simulink model "DrivetrainEv"  (R2020a)
settings: Solver=VariableStepAuto  StartTime=0.0  StopTime=2474  RelTol=1e-3  EnableMultiTasking=on
model workspace (MAT data in the model file):
  Af = 2.27
  Bx = 10
  Cd = 0.28
  Cl = 0.1
  Cpm = 0.1
  Cx = 1.65
  Dx = 1
  Ex = 0.01
  FZMAX = 6570
  FZMIN = 0
  Fc = 500
  FsbF = [-700000 -7000 -700 0 700 7000 700000]
  FsbR = [-700000 -7000 -700 0 700 7000 700000]
  FskF = [-8928.57142857 -178.571428571 0 357.142857143 535.714285714 9285.71428571]
  FskR = [-5357.14285714 -107.142857143 0 214.285714286 321.428571429 5571.42857143]
  Iyy = 3000
  Iyy_Whl = 0.8
  J = 0.01
  Jd = 0.025
  Jmotor = 0.023
  Jw1 = 0.01
  Jw2 = 0.01
  Lrel = 0.15
  Mass = 235.45
  NF = 2
  NR = 2
  Ndiff = 7.94
  Ndisks = 4
  Pabs = 101325
  Re = 0.203
  Reff_LSD = 0.2
  Rm = 0.15
  T = 273
  UNLOADED_RADIUS = 0.206
  VXLOW = 2
  aMy = 0.01
  a_CG = 1.188
  alphaMy = 0
  b = Simulink.Parameter
  b.Value = 400
  b.DataType = 'auto'
  b.Dimensions = [1 1]
  b1 = 100
  bMy = 0
  b_CG = 1.512
  b_J = 0.001
  bd = 0.001
  betaMy = 1
  br = 0.001
  bw1 = 0.001
  bw2 = 0.001
  cMy = 0
  disk_abore = 0.05
  domega_o = 0
  dw = [0 10 20 40 60 80 100]
  dzdotsF = [-10 -1 -0.1 0 0.1 1 10]
  dzdotsR = [-10 -1 -0.1 0 0.1 1 10]
  dzsF = [-0.005 -0.0001 0 0.2 0.2001 0.2051]
  dzsR = [-0.005 -0.0001 0 0.2 0.2001 0.2051]
  g = 9.81
  h = 0.5
  k = Simulink.Parameter
  k.Value = 10000
  k.DataType = 'auto'
  k.Dimensions = [1 1]
  k1 = 50000
  kappamax = 1.5
  lam_x = 1
  mu_kinetic = 0.35
  mu_static = 0.45
  muc = [0.16 0.13 0.115 0.11 0.105 0.1025 0.10125]
  num_pads = 2
  omega1_c = 3000
  omega_c = Simulink.Parameter
  omega_c.Value = 100
  omega_c.DataType = 'auto'
  omega_c.Dimensions = [1 1]
  omega_o = 0
  omega_o_J = 0
  omegao = 0
  omegaw1o = 0
  omegaw2o = 0
  press = 234400
  q_o = 0
  tauC_LSD = 0.01
  theta_o = 0
  theta_o_Veh = 0
  wc_shaft = Simulink.Parameter
  wc_shaft.Value = 0.1
  wc_shaft.DataType = 'auto'
  wc_shaft.Dimensions = [1 1]
  x_o = 0
  xdot_o = 0
  z_o = -0.35
  zdot_o = 0
libraries: autolibsharedcoupling x7, autolibpowerinfoutils x6, autolibshareddiff x4, autolibshared x3, autolibcoupling x1
(part 1 of 3)
settings Model: ModifiedByFormat=The MathWorks, Inc.  SimulationMode=rapid-accelerator  PauseTimes=10  Creator=The MathWorks, Inc.  LastModifiedBy=The MathWorks, Inc.
settings SolverCC: DecoupledContinuousIntegration=on  MinimalZcImpactIntegration=on
settings DataIOCC: DSMLogging=off  ReturnWorkspaceOutputs=off
settings DebuggingCC: MergeDetectMultiDrivingBlocksExec=none  PregeneratedLibrarySubsystemCodeDiagnostic=none  ArithmeticOperatorsInVariantConditions=warning
settings ModelReferenceCC: PropagateSignalLabelsOutOfModel=off
settings SFSimCC: SimUseLocalCustomCode=off
settings RTWCC: RTWUseLocalCustomCode=off
settings CodeAppCC: StateflowObjectComments=on
settings GRTTargetCC: TargetLangStandard=C89/C90 (ANSI)
settings ConfigComp: CovMetricSettings=dsw  CovHtmlReporting=on  CovSaveCumulativeToWorkspaceVar=on  CovSaveSingleToWorkspaceVar=on  CovShowResultsExplorer=off  CovExternalEMLEnable=off
settings SimscapeCC: SimscapeNormalizeSystem=off

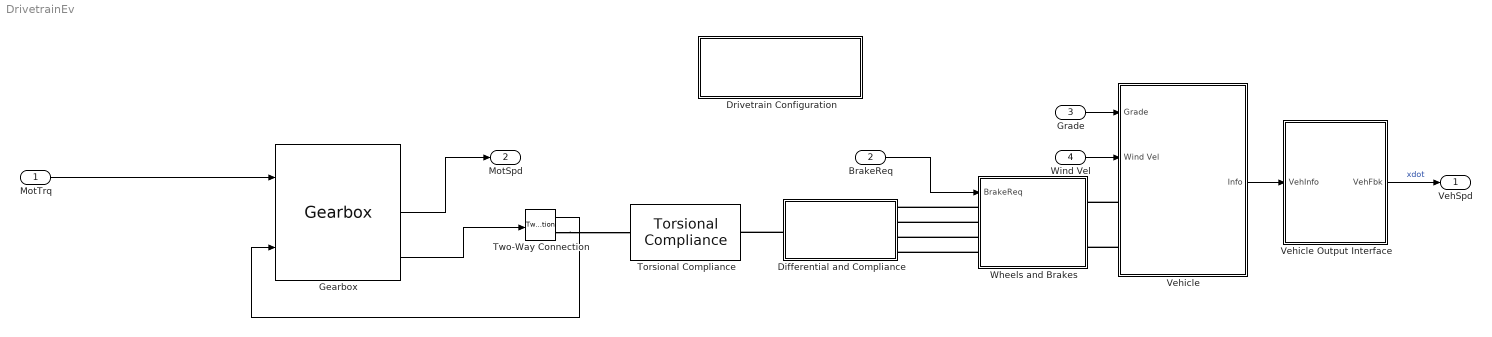
== system DrivetrainEv ==
  MotTrq : Inport
  BrakeReq : Inport  Port=2
  Grade : Inport  Port=3
  Wind Vel : Inport  Port=4
  Differential and Compliance : Subsystem  Variant=on  VariantControlMode=Label  LabelModeActiveChoice=1
  Drivetrain Configuration : Subsystem  mask(Drivetrain Configuration){drivetrainMode=Rear Wheel Drive}
      mask prompts: drivetrainMode "Drivetrain Mode"
      mask help: Use this block to configure the dirvetrain mode.
      settings: AttributesFormatString=Active Mode: %<drivetrainMode>
      mask TypeOptions drivetrainMode: Front Wheel Drive | Rear Wheel Drive | All Wheel Drive
      mask Callback drivetrainMode:
      | switch get_param(gcb,'drivetrainMode')
      |     case 'Front Wheel Drive'
      |         set_param([bdroot '/Differential and Compliance'],'OverrideUsingVariant','0')
      |     case 'Rear Wheel Drive'
      |         set_param([bdroot '/Differential and Compliance'],'OverrideUsingVariant','1')
      |     case 'All Wheel Drive'
      |         set_param([bdroot '/Differential and Compliance'],'OverrideUsingVariant','2')
      |     otherwise
      |         set_param([bdroot '/Differential and Compliance'],'OverrideUsingVariant','0')
      | end
      mask Display: disp('Double click to configure drivetrain')
  Gearbox : autolibcoupling/Gearbox  port_config=Simulink  input_config=Torque input - velocity output  DiffEffModelPopup=Constant  InterpMethod=Flat  dirSwitch=on  extTamb=off  N=9/40  J1=.023  J2=.023  b1=0  b2=0  theta1_o=0  w1_o=0  eta=1  eta_tbl=reshape([0.64 0.76 0.8 0.81 0.83 0.84 0.84 0.56 0.73 0.78 0.8 0.83 0.84 0.84 0.54 0.71 0.77 0.8 0.82 0.84 0.84 0.53 0.71 0.77 0.8 0.83 0.84 0.84 0.51 0.71 0.77 0.8 0.83 0.84 0.85 0.52 0.7 0.77 0.8 0.83 0.84 0.85 0.51 0.71 0.76 0.79 0.83 0.84 0.85 0.5 0.69 0.76 0.79 0.82 0.84 0.85 0.45 0.68 0.75 0.78 0.82 0.84 0.85 0.43 0.67 0.74 0.78 0.81 0.83 0.84 0.38 0.63 0.71 0.75 0.8 0.82 0.83 0.81 0.86 0.88 0.89 0.89 0.89 0.9 0.77 0.85 0.87 0.88 0.89 0.9 0.9 0.72 0.82 0.86 0.87 0.88 0.89 0.9 0.68 0.8 0.84 0.86 0.88 0.89 0.89 0.67 0.8 0.84 0.86 0.88 0.89 0.9 0.67 0.8 0.84 0.86 0.88 0.89 0.9 0.65 0.8 0.84 0.86 0.88 0.89 0.9 0.64 0.79 0.83 0.86 0.88 0.89 0.9 0.63 0.78 0.83 0.86 0.88 0.89 0.9 0.59 0.76 0.82 0.85 0.87 0.89 0.9 0.53 0.73 0.8 0.83 0.86 0.88 0.89], 7, 11, 2)  Trq_bpts=[25, 50, 75, 100, 150, 200, 250]  omega_bpts=[52.4 78.5 105 131 157 183 209 262 314 419 524]  Temp_bpts=[290 358]  Tamb=297.15  blkID=0
      settings: SourceProductBaseCode=PW
  Torsional Compliance : autolibsharedcoupling/Torsional Compliance  port_config=Two-way connection  extInfo=off  k=1e4  b=1e2  theta_o=0  domega_o=0  omega_c=3000  blkID=0  aMode=1
      settings: SourceProductBaseCode=PW,MT,VE,VP
  Two-Way Connection : TwoWayConnection
  Vehicle : Subsystem
  Vehicle Output Interface : Subsystem
  Wheels and Brakes : Subsystem  VariantControl=0
  VehSpd : Outport  VectorParamsAs1DForOutWhenUnconnected=off
  MotSpd : Outport  Port=2  VectorParamsAs1DForOutWhenUnconnected=off  BusOutputAsStruct=on
  wires:
  BrakeReq/1 -> Wheels and Brakes/1(BrakeReq)
  Vehicle/1(Info) -> Vehicle Output Interface/1(VehInfo)
  Vehicle Output Interface/1(VehFbk) -> VehSpd/1  "xdot"
  Wind Vel/1 -> Vehicle/2(Wind Vel)
  Grade/1 -> Vehicle/1(Grade)
  MotTrq/1 -> Gearbox/1
  Gearbox/2 -> MotSpd/1
  Gearbox/3 -> Two-Way Connection/1
  Two-Way Connection/1 -> Gearbox/2
  connections:
  Wheels and Brakes/LConn1 -- Differential and Compliance/RConn1
  Wheels and Brakes/LConn2 -- Differential and Compliance/RConn2
  Wheels and Brakes/LConn3 -- Differential and Compliance/RConn3
  Wheels and Brakes/LConn4 -- Differential and Compliance/RConn4
  Vehicle/LConn1 -- Wheels and Brakes/RConn1
  Vehicle/LConn2 -- Wheels and Brakes/RConn2
  Differential and Compliance/LConn1 -- Torsional Compliance/RConn1
  Two-Way Connection/RConn1 -- Torsional Compliance/LConn1

== system DrivetrainEv/Differential and Compliance ==
  All Wheel Drive : Subsystem  VariantControl=2
  Front Wheel Drive : Subsystem  VariantControl=0
  Rear Wheel Drive : Subsystem  VariantControl=1
  D : PMIOPort  Side=Left
  FA1 : PMIOPort  Port=2  Side=Right
  FA2 : PMIOPort  Port=3  Side=Right
  RA1 : PMIOPort  Port=4  Side=Right
  RA2 : PMIOPort  Port=5  Side=Right

== system DrivetrainEv/Drivetrain Configuration ==

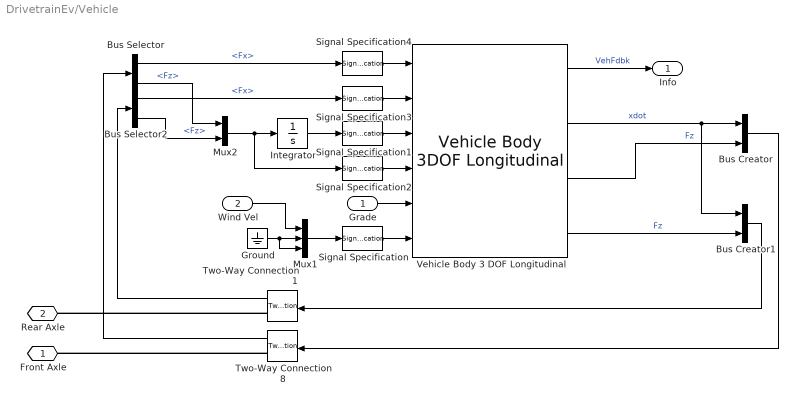
== system DrivetrainEv/Vehicle ==
  Grade : Inport  Unit=deg
  Wind Vel : Inport  Port=2  Unit=m/s
  Bus Creator : BusCreator  Inputs=2
  Bus Creator1 : BusCreator  Inputs=2
  Bus Selector : BusSelector  OutputSignals=Fx,Fz
  Bus Selector2 : BusSelector  OutputSignals=Fx,Fz
  Ground : Ground
  Integrator : Integrator
  Mux1 : Mux  Inputs=3
  Mux2 : Mux  Inputs=2
  Signal Specification : SignalSpecification  Unit=m/s
  Signal Specification1 : SignalSpecification  Unit=m
  Signal Specification2 : SignalSpecification  Unit=m/s
  Signal Specification3 : SignalSpecification  Unit=N
  Signal Specification4 : SignalSpecification  Unit=N
  Two-Way Connection1 : TwoWayConnection
  Two-Way Connection8 : TwoWayConnection
  Vehicle Body 3 DOF Longitudinal : autolibshared/Vehicle Body 3DOF Longitudinal  VariantControl=SL  groundType=Axle displacement, velocity  aMode=1  extFMode=off  extMMode=off  extTamb=off  NF=NF  NR=NR  m=Mass  a=a_CG  b=b_CG  h=h  Cd=Cd  Af=Af  x_o=x_o  xdot_o=xdot_o  Cl=Cl  z_o=z_o  zdot_o=zdot_o  Iyy=Iyy  Cpm=Cpm  theta_o=theta_o_Veh  q_o=q_o  FskF=FskF  dzsF=dzsF  FsbF=FsbF  dzdotsF=dzdotsF  FskR=FskR  dzsR=dzsR  FsbR=FsbR  dzdotsR=dzdotsR  Pabs=Pabs  T=T  g=g  blkID=0
      settings: SourceProductBaseCode=PW,MT,VE,VP
  Front Axle : PMIOPort  Side=Left
  Rear Axle : PMIOPort  Port=2  Side=Left
  Info : Outport  VectorParamsAs1DForOutWhenUnconnected=off
  wires:
  Two-Way Connection1/1 -> Bus Selector2/1
  Bus Selector2/2 -> Mux2/2  "<Fz>"
  Bus Selector2/1 -> Signal Specification3/1  "<Fx>"
  Bus Selector/2 -> Mux2/1  "<Fz>"
  Bus Selector/1 -> Signal Specification4/1  "<Fx>"
  Bus Creator1/1 -> Two-Way Connection1/1
  Bus Creator/1 -> Two-Way Connection8/1
  Signal Specification4/1 -> Vehicle Body 3 DOF Longitudinal/1
  Signal Specification3/1 -> Vehicle Body 3 DOF Longitudinal/2
  Signal Specification2/1 -> Vehicle Body 3 DOF Longitudinal/4
  Signal Specification1/1 -> Vehicle Body 3 DOF Longitudinal/3
  Signal Specification/1 -> Vehicle Body 3 DOF Longitudinal/6
  Grade/1 -> Vehicle Body 3 DOF Longitudinal/5
  Wind Vel/1 -> Mux1/1
  Integrator/1 -> Signal Specification1/1
  Mux2/1 -> Signal Specification2/1, Integrator/1
  Vehicle Body 3 DOF Longitudinal/4 -> Bus Creator1/2  "Fz"
  Mux1/1 -> Signal Specification/1
  Ground/1 -> Mux1/3, Mux1/2
  Vehicle Body 3 DOF Longitudinal/1 -> Info/1  "VehFdbk"
  Two-Way Connection8/1 -> Bus Selector/1
  Vehicle Body 3 DOF Longitudinal/2 -> Bus Creator/1, Bus Creator1/1  "xdot"
  Vehicle Body 3 DOF Longitudinal/3 -> Bus Creator/2  "Fz"
  connections:
  Two-Way Connection1/RConn1 -- Rear Axle/RConn1
  Two-Way Connection8/RConn1 -- Front Axle/RConn1

== system DrivetrainEv/Vehicle Output Interface ==
  VehInfo : Inport
  Bus Selector1 : BusSelector  OutputSignals=BdyFrm.Cg.Vel.xdot
  VehFbk : Outport  VectorParamsAs1DForOutWhenUnconnected=off
  wires:
  Bus Selector1/1 -> VehFbk/1  "<xdot>"
  VehInfo/1 -> Bus Selector1/1
